simulink model "MASH20_system_integration"  (R2024a)
settings: Solver=ode45  StartTime=0.0  StopTime=1  MaxStep=Ts/10  EnableMultiTasking=on
PreLoadFcn:
  | s0=sprintf('===========================================================================');disp(s0)
  | s1=sprintf('= Created by Bader Almutair bmutairi@kacst.edu.sa                         =');disp(s1)
  | s2=sprintf('= Date 12/11/2014                                                         =');disp(s2)
  | s3=sprintf('= Refer to the PhD thesis Ch4,P.55                                        =');disp(s3)
  | s4=sprintf('===========================================================================');disp(s4)
values from neighbouring files (symbols this model uses):
  AA = AA_design*(mismatch_lower_limit + rand_range*rand)    [simon_test.m]    (also in testPSD_simulink.m)
  b = b_design*(0.8 + (1.2 - 0.8) * rand)    [D2_parameter_mapping.m]    (also in simon_test.m = b_design*(mismatch_lower_limit + rand_range*rand); testPSD_simulink.m = b_design*(mismatch_lower_limit + rand_range*rand))
  d0 = d0_design*(mismatch_lower_limit + rand_range*rand)    [simon_test.m]    (also in testPSD_simulink.m)
  enoise = 10e-9    (= 1e-08)    [simon_test.m]    (also in testPSD_simulink.m)
  epsilon = 8.854e-12    [population_score_c2d.m]    (also in simon_test.m; testPSD_c2d.m; testPSD_simulink.m)
  Finput = F_resolution*128    (= 260.4140625)    [new_generation_coeff.m]    (also in simon_test.m; testPSD_simulink.m)
  k = k_design*(0.8 + (1.2 - 0.8) * rand)    [D2_parameter_mapping.m]    (also in log2_linear_taylor.m = floor(log2(x)); population_score.m = floor(log2(real(Y3).^2 + imag(Y3).^2)); population_score_c2d.m = floor(log2(Y3)); simon_test.m = k_design*(mismatch_lower_limit + rand_range*rand))
  Kfb = Kfb_design*(0.8 + (1.2 - 0.8) * rand)    [D2_parameter_mapping.m]    (also in simon_test.m = 0.5*epsilon*AA*(Vfeedback^2)/(d0^2); testPSD_simulink.m = 0.5*epsilon*AA*(Vfeedback^2)/(d0^2))
  Kpo = Kpo_design*(0.8 + (1.2 - 0.8) * rand)    [D2_parameter_mapping.m]    (also in simon_test.m = Kpo_design*(mismatch_lower_limit + rand_range*rand); testPSD_simulink.m = Kpo_design*(mismatch_lower_limit + rand_range*rand))
  Lfactor = Vfeedback/d0    [simon_test.m]    (also in testPSD_simulink.m)
  m = m_design*(0.8 + (1.2 - 0.8) * rand)    [D2_parameter_mapping.m]    (also in simon_test.m = m_design*(mismatch_lower_limit + rand_range*rand); testPSD_simulink.m = m_design*(mismatch_lower_limit + rand_range*rand))
  Ts = 1/Fs    (= 7.50007500075e-06)    [new_generation_coeff.m]    (also in simon_test.m; simple_fft_test.m = 1/F; testPSD_c2d.m; testPSD_simulink.m)
  Vfeedback = Vfeedback_design*(mismatch_lower_limit + rand_range*rand)    [simon_test.m]    (also in testPSD_simulink.m)
  x = linspace(min(a4), max(a4), 100)    [D2_parameter_mapping.m]    (also in log2_linear_taylor.m = 1e-10; simon_test.m = 0.9; testPSD_simulink.m = 0.9)
libraries: simulink_extras x2, dspsigops x1
settings Model: Creator=Administrator  LastModifiedBy=Simon
settings SolverCC: AlgebraicLoopSolver=TrustRegion
settings DataIOCC: LimitDataPoints=on  SaveFormat=Array  SignalLoggingSaveFormat=ModelDataLogs  ReturnWorkspaceOutputs=off
settings OptimizationCC: ReuseModelBlockBuffer=off  ExpressionDepthLimit=2147483647  LifeSpan=inf
settings DebuggingCC: UnderspecifiedInitializationDetection=Classic  MergeDetectMultiDrivingBlocksExec=none  SolverPrmCheckMsg=warning  FcnCallInpInsideContextMsg=warning  UnconnectedInputMsg=warning  UnconnectedOutputMsg=warning  UnconnectedLineMsg=warning  StateNameClashWarn=warning  SFUnexpectedBacktrackingDiag=warning  SFNoUnconditionalDefaultTransitionDiag=warning  SFExecutionAtInitializationDiag=none  ArithmeticOperatorsInVariantConditions=warning
settings HardwareCC: ProdBitPerPointer=32  ProdBitPerSizeT=32  ProdBitPerPtrDiffT=32  ProdLargestAtomicFloat=None  ProdIntDivRoundTo=Undefined  ProdEndianess=Unspecified  ProdWordSize=32  ProdHWDeviceType=32-bit Generic
settings ModelReferenceCC: PropagateSignalLabelsOutOfModel=off
settings SFSimCC: SimUseLocalCustomCode=off  CustomCodeUndefinedFunction=UseInterfaceOnly
settings RTWCC: RTWUseLocalCustomCode=off  GPUComputeCapability=3.5
settings CodeAppCC: StateflowObjectComments=on
settings GRTTargetCC: TargetLangStandard=C89/C90 (ANSI)  CombineOutputUpdateFcns=off  GRTInterface=on
settings ConfigComp: CovMetricSettings=dw  CovSaveCumulativeToWorkspaceVar=on  CovSaveSingleToWorkspaceVar=on  CovExternalEMLEnable=off

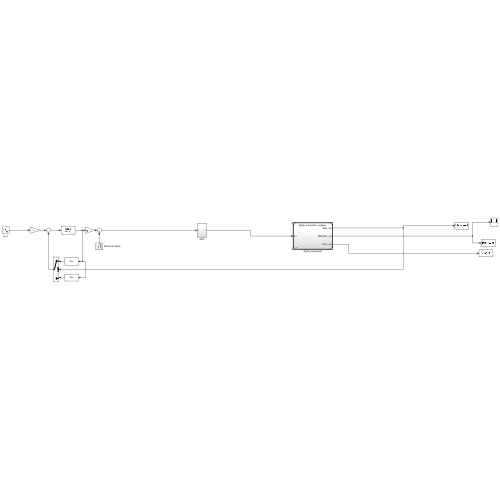
[thumbnail: Simulink's stored preview of the top-level diagram]
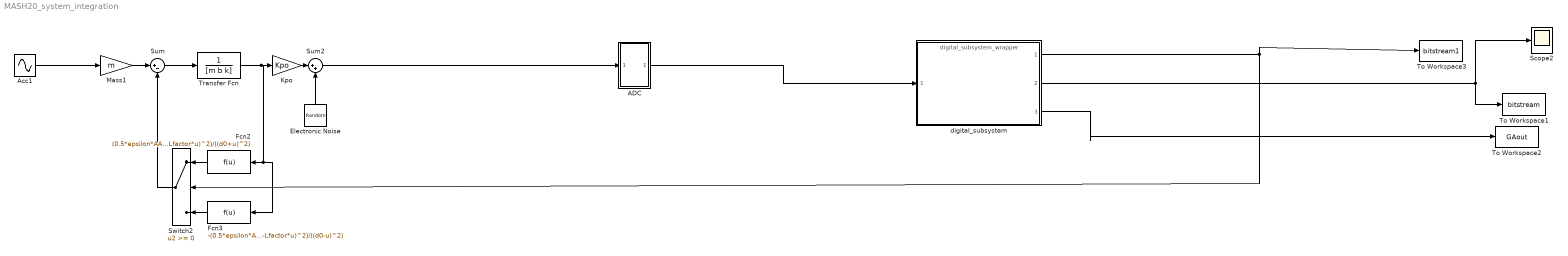
== system MASH20_system_integration ==
  ADC : Subsystem
  Acc1 : Sin  Amplitude=(Kfb/m)*x  Frequency=Finput*2*pi  SampleTime=0
  Electronic Noise : RandomNumber  Variance=(enoise*sqrt(5/Ts))^2  Seed=432  SampleTime=Ts
  Fcn2 : Fcn  Expr=(0.5*epsilon*AA*(Vfeedback+Lfactor*u)^2)/((d0+u)^2)
  Fcn3 : Fcn  Expr=-(0.5*epsilon*AA*(Vfeedback-Lfactor*u)^2)/((d0-u)^2)
  Kpo : Gain  Gain=Kpo
  Mass1 : Gain  Gain=m
  Scope2 : Scope
  Sum : Sum  Inputs=|+-
  Sum2 : Sum  Inputs=|++
  Switch2 : Switch  SaturateOnIntegerOverflow=off  InputSameDT=off
  To Workspace1 : ToWorkspace  VariableName=bitstream  SampleTime=Ts
  To Workspace2 : ToWorkspace  VariableName=GAout  SampleTime=Ts
  To Workspace3 : ToWorkspace  VariableName=bitstream1  SampleTime=Ts
  Transfer Fcn : TransferFcn  Denominator=[m b k]
  digital_subsystem : ModelReference  ModelNameDialog=digital_subsystem_wrapper  SimulationMode=Normal  ModelReferenceVersion=24.5
  wires:
  Transfer Fcn/1 -> Fcn3/1, Fcn2/1, Kpo/1
  Sum/1 -> Transfer Fcn/1
  Mass1/1 -> Sum/1
  Fcn2/1 -> Switch2/1
  Fcn3/1 -> Switch2/3
  Switch2/1 -> Sum/2
  Kpo/1 -> Sum2/1
  Electronic Noise/1 -> Sum2/2
  Acc1/1 -> Mass1/1
  digital_subsystem/1 -> Switch2/2, To Workspace3/1
  digital_subsystem/2 -> To Workspace1/1, Scope2/1
  digital_subsystem/3 -> To Workspace2/1
  Sum2/1 -> ADC/1(In1)
  ADC/1(Out1) -> digital_subsystem/1

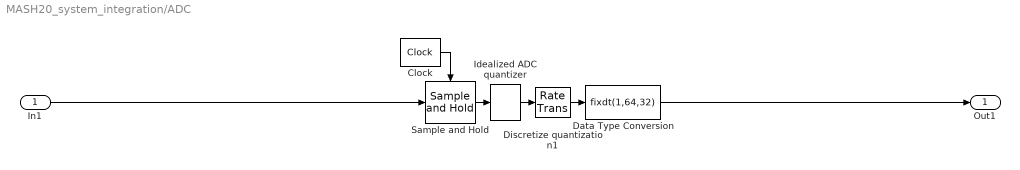
== system MASH20_system_integration/ADC ==
  In1 : Inport
  Clock : simulink_extras/Flip Flops/Clock  period=Ts
  Data Type Conversion : DataTypeConversion  OutDataTypeStr=fixdt(1,64,32)  SaturateOnIntegerOverflow=off  RndMeth=Floor
  Discretize quantization1 : RateTransition  OutPortSampleTime=Ts
  Idealized ADC quantizer : simulink_extras/Additional Discrete/Idealized ADC quantizer  NumberOfConverterBits=12  Vmin=-2.5  Vmax=2.5  OutputDataType=double  OutputNegativeValues=on
  Sample and Hold : dspsigops/Sample and Hold  trig=Rising edge  initCond=0  latchinput=off
  Out1 : Outport
  wires:
  Discretize quantization1/1 -> Data Type Conversion/1
  Idealized ADC quantizer/1 -> Discretize quantization1/1
  Clock/1 -> Sample and Hold/Trigger
  In1/1 -> Sample and Hold/1
  Data Type Conversion/1 -> Out1/1
  Sample and Hold/1 -> Idealized ADC quantizer/1
